simulink model "Q3"  (R2021b)
settings: Solver=ode1  StartTime=0.0  StopTime=15  FixedStep=100e-6  RelTol=1e-3
settings Model: Creator=yyx  LastModifiedBy=Divin

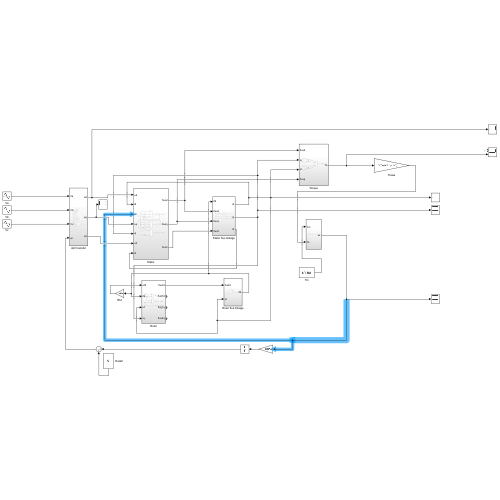
[thumbnail: Simulink's stored preview of the top-level diagram]
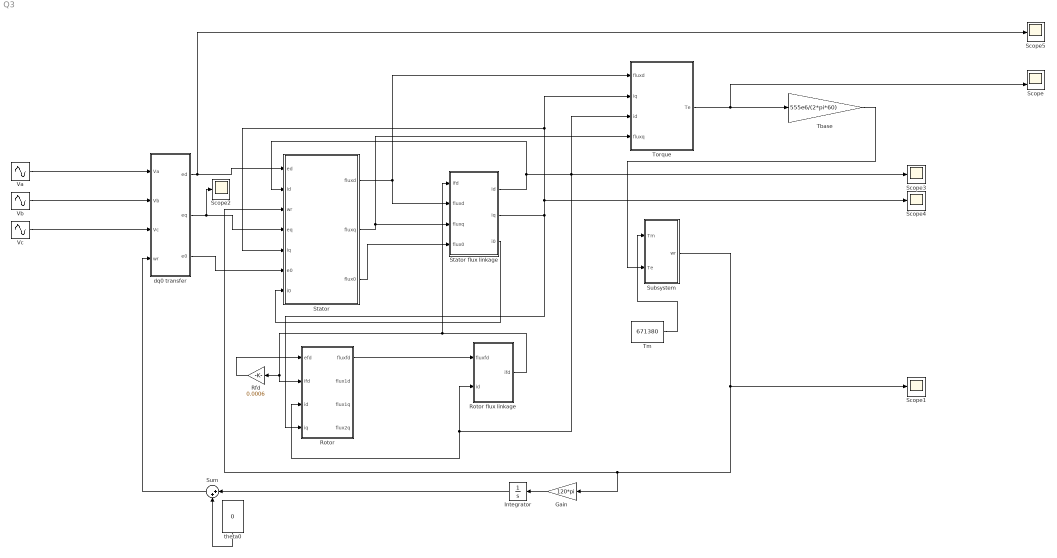
== system Q3 ==
  Gain : Gain  Gain=120*pi
  Integrator : Integrator
  Rfd : Gain  Gain=0.0006
  Rotor : Subsystem
  Rotor flux linkage : Subsystem
  Scope : Scope  NumInputPorts=2
  Scope{1..5} (5 alike) : Scope
  Stator : Subsystem
  Stator flux linkage : Subsystem
  Subsystem : Subsystem
  Sum : Sum  Inputs=|++
  Tbase : Gain  Gain=555e6/(2*pi*60)
  Tm : Constant  Value=671380
  Torque : Subsystem
  Va : Sin  Frequency=2*pi*60  Samples=2*pi/(60*2*pi*15)  SampleTime=0
  Vb : Sin  Frequency=2*pi*60  Phase=-2*pi/3  SampleTime=0
  Vc : Sin  Frequency=2*pi*60  Phase=2*pi/3  SampleTime=0
  dq0 transfer : Subsystem
  theta0 : Constant  Value=0
  wires:
  Va/1 -> dq0 transfer/1(Va)
  Vb/1 -> dq0 transfer/2(Vb)
  Vc/1 -> dq0 transfer/3(Vc)
  dq0 transfer/1(ed) -> Scope5/1, Stator/1(ed)
  dq0 transfer/2(eq) -> Stator/4(eq), Scope2/1
  Stator flux linkage/1(id) -> Stator/2(id), Rotor/3(id), Rotor flux linkage/2(id), Torque/3(id), Scope3/1
  Stator flux linkage/2(iq) -> Torque/2(iq), Stator/5(iq), Scope4/1, Rotor/4(iq)
  dq0 transfer/3(e0) -> Stator/6(e0)
  Stator flux linkage/3(i0) -> Stator/7(i0)
  Subsystem/1(wr) -> Gain/1, Stator/3(wr), Scope1/1
  Stator/1(fluxd) -> Stator flux linkage/2(fluxd), Torque/1(fluxd)
  Stator/2(fluxq) -> Torque/4(fluxq), Stator flux linkage/3(fluxq)
  Stator/3(flux0) -> Stator flux linkage/4(flux0)
  Rotor flux linkage/1(ifd) -> Rfd/1, Rotor/2(ifd), Stator flux linkage/1(ifd)
  Rotor/1(fluxfd) -> Rotor flux linkage/1(fluxfd)
  Rfd/1 -> Rotor/1(efd)
  Torque/1(Te) -> Scope/2, Tbase/1
  Tm/1 -> Subsystem/1(Tm)
  Integrator/1 -> Sum/1
  Tbase/1 -> Subsystem/2(Te)
  Gain/1 -> Integrator/1
  Sum/1 -> dq0 transfer/4(wr)
  theta0/1 -> Sum/2

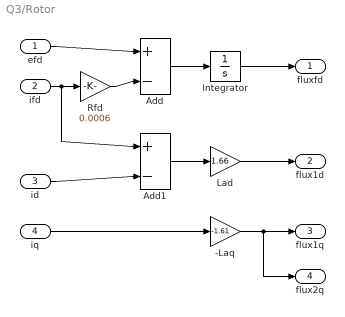
== system Q3/Rotor ==
  efd : Inport
  ifd : Inport  Port=2
  id : Inport  Port=3
  iq : Inport  Port=4
  -Laq : Gain  Gain=-1.61
  Add : Sum  Inputs=+|-
  Add1 : Sum  Inputs=+|-
  Integrator : Integrator
  Lad : Gain  Gain=1.66
  Rfd : Gain  Gain=0.0006
  fluxfd : Outport
  flux1d : Outport  Port=2
  flux1q : Outport  Port=3
  flux2q : Outport  Port=4
  wires:
  ifd/1 -> Add1/1, Rfd/1
  efd/1 -> Add/1
  Integrator/1 -> fluxfd/1
  Add/1 -> Integrator/1
  Rfd/1 -> Add/2
  id/1 -> Add1/2
  Add1/1 -> Lad/1
  Lad/1 -> flux1d/1
  iq/1 -> -Laq/1
  -Laq/1 -> flux2q/1, flux1q/1

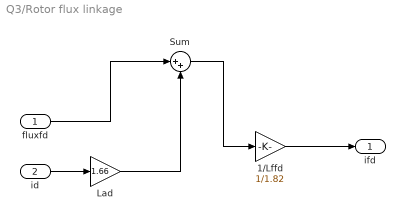
== system Q3/Rotor flux linkage ==
  fluxfd : Inport
  id : Inport  Port=2
  1/Lffd : Gain  Gain=1/1.82
  Lad : Gain  Gain=1.66
  Sum : Sum  Inputs=|++
  ifd : Outport
  wires:
  id/1 -> Lad/1
  Lad/1 -> Sum/2
  1/Lffd/1 -> ifd/1
  fluxfd/1 -> Sum/1
  Sum/1 -> 1/Lffd/1

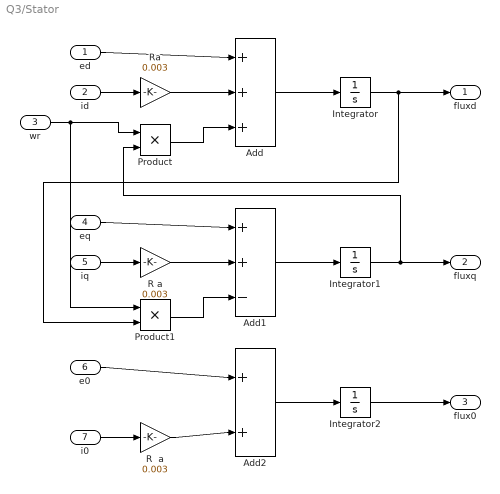
== system Q3/Stator ==
  ed : Inport
  id : Inport  Port=2
  wr : Inport  Port=3
  eq : Inport  Port=4
  iq : Inport  Port=5
  e0 : Inport  Port=6
  i0 : Inport  Port=7
  Add : Sum  Inputs=+|+|+
  Add1 : Sum  Inputs=+|+|-
  Add2 : Sum  Inputs=+|+
  Integrator : Integrator
  Integrator1 : Integrator
  Integrator2 : Integrator
  Product : Product
  Product1 : Product
  R  a : Gain  Gain=0.003
  R a : Gain  Gain=0.003
  Ra : Gain  Gain=0.003
  fluxd : Outport
  fluxq : Outport  Port=2
  flux0 : Outport  Port=3
  wires:
  wr/1 -> Product1/1, Product/1
  R a/1 -> Add1/2
  Integrator1/1 -> fluxq/1, Product/2
  Product/1 -> Add/3
  iq/1 -> R a/1
  Integrator/1 -> fluxd/1, Product1/2
  ed/1 -> Add/1
  id/1 -> Ra/1
  Product1/1 -> Add1/3
  Add1/1 -> Integrator1/1
  Add/1 -> Integrator/1
  Ra/1 -> Add/2
  eq/1 -> Add1/1
  e0/1 -> Add2/1
  i0/1 -> R  a/1
  R  a/1 -> Add2/2
  Add2/1 -> Integrator2/1
  Integrator2/1 -> flux0/1

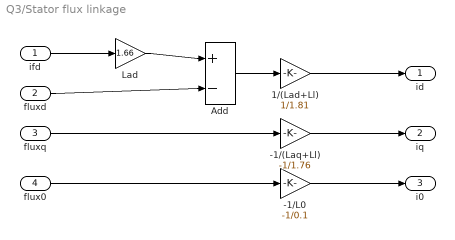
== system Q3/Stator flux linkage ==
  ifd : Inport
  fluxd : Inport  Port=2
  fluxq : Inport  Port=3
  flux0 : Inport  Port=4
  -1/(Laq+Ll) : Gain  Gain=-1/1.76
  -1/L0 : Gain  Gain=-1/0.1
  1/(Lad+Ll) : Gain  Gain=1/1.81
  Add : Sum  Inputs=+|-
  Lad : Gain  Gain=1.66
  id : Outport
  iq : Outport  Port=2
  i0 : Outport  Port=3
  wires:
  -1/L0/1 -> i0/1
  fluxd/1 -> Add/2
  -1/(Laq+Ll)/1 -> iq/1
  1/(Lad+Ll)/1 -> id/1
  Lad/1 -> Add/1
  Add/1 -> 1/(Lad+Ll)/1
  ifd/1 -> Lad/1
  fluxq/1 -> -1/(Laq+Ll)/1
  flux0/1 -> -1/L0/1

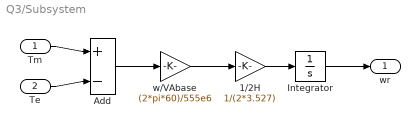
== system Q3/Subsystem ==
  Tm : Inport
  Te : Inport  Port=2
  1/2H : Gain  Gain=1/(2*3.527)
  Add : Sum  Inputs=+|-
  Integrator : Integrator
  w/VAbase : Gain  Gain=(2*pi*60)/555e6
  wr : Outport
  wires:
  Add/1 -> w/VAbase/1
  Tm/1 -> Add/1
  w/VAbase/1 -> 1/2H/1
  Integrator/1 -> wr/1
  Te/1 -> Add/2
  1/2H/1 -> Integrator/1

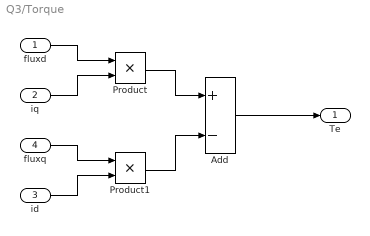
== system Q3/Torque ==
  fluxd : Inport
  iq : Inport  Port=2
  id : Inport  Port=3
  fluxq : Inport  Port=4
  Add : Sum  Inputs=+|-
  Product : Product
  Product1 : Product
  Te : Outport
  wires:
  fluxq/1 -> Product1/1
  iq/1 -> Product/2
  fluxd/1 -> Product/1
  Product1/1 -> Add/2
  Add/1 -> Te/1
  id/1 -> Product1/2
  Product/1 -> Add/1

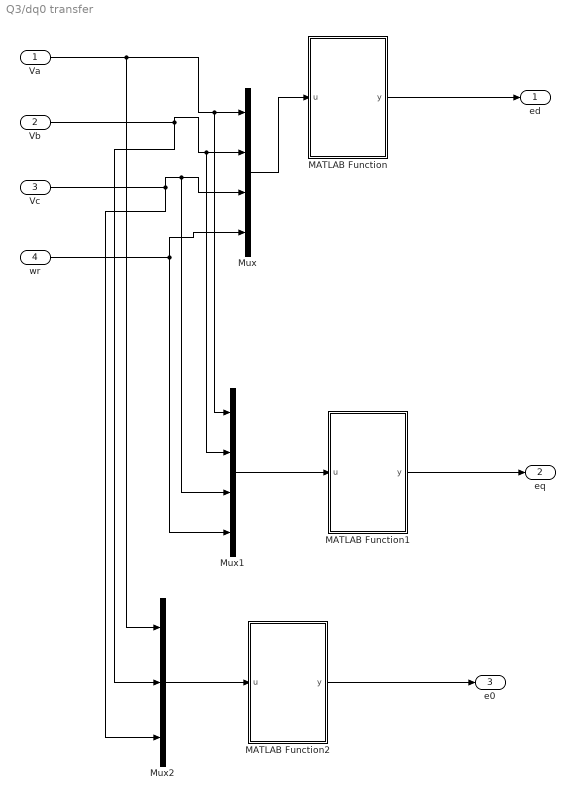
== system Q3/dq0 transfer ==
  Va : Inport
  Vb : Inport  Port=2
  Vc : Inport  Port=3
  wr : Inport  Port=4
  MATLAB Function : MATLAB Function  TreatAsAtomicUnit=on
  MATLAB Function1 : MATLAB Function  TreatAsAtomicUnit=on
  MATLAB Function2 : MATLAB Function  TreatAsAtomicUnit=on
  Mux : Mux
  Mux1 : Mux
  Mux2 : Mux  Inputs=3
  ed : Outport
  eq : Outport  Port=2
  e0 : Outport  Port=3
  wires:
  MATLAB Function/1(y) -> ed/1
  Va/1 -> Mux/1, Mux1/1, Mux2/1
  Vc/1 -> Mux1/3, Mux/3, Mux2/3
  wr/1 -> Mux/4, Mux1/4
  Mux/1 -> MATLAB Function/1(u)
  MATLAB Function2/1(y) -> e0/1
  MATLAB Function1/1(y) -> eq/1
  Mux2/1 -> MATLAB Function2/1(u)
  Mux1/1 -> MATLAB Function1/1(u)
  Vb/1 -> Mux1/2, Mux/2, Mux2/2

== matlab function Q3/dq0 transfer/MATLAB Function1 ==
  data: u input; y output
function y = fcn(u)

y = (2/3)*(-sin(u(4))*u(1)-sin(u(4)-2*pi/3)*u(2)-sin(u(4)+2*pi/3)*u(3));

== matlab function Q3/dq0 transfer/MATLAB Function ==
  data: u input; y output
function y = fcn(u)

y = (2/3)*(cos(u(4))*u(1)+cos(u(4)-2*pi/3)*u(2)+cos(u(4)+2*pi/3)*u(3));

== matlab function Q3/dq0 transfer/MATLAB Function2 ==
  data: u input; y output
function y = fcn(u)

y = (1/3)*(u(1)+u(2)+u(3));
